simulink model "testmodel"  (R2019b)
settings: Solver=VariableStepAuto  StartTime=0.0  StopTime=10.0  RelTol=1e-3
settings Model: Creator=Alexander  LastModifiedBy=Alexander

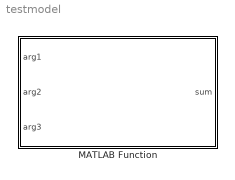
== system testmodel ==
  MATLAB Function : MATLAB Function  TreatAsAtomicUnit=on

== matlab function testmodel/MATLAB Function ==
  data: arg1 input; sum output; arg2 input; arg3 input
function sum  = sum_of_three(arg1,arg2,arg3)
% the function returns the sum of three input args

% default value of arg3
switch nargin
    case 0
        arg1=0;
        arg2=0;
        arg3=0;
    case 1
        arg2=0;
        arg3=0;
    case 2
        arg3=0;
end
    
sum = arg1 + arg2 + arg3;

end
